simulink model "robotarm_A12"  (R2018b)
settings: Solver=FixedStepAuto  StartTime=0.0  StopTime=options.T_train  RelTol=1e-3  AbsTol=1e-6
undefined symbols (not defined in the file or in its folder): options
libraries: neural x132, simulink x2
(part 6 of 6)

== system robotarm_A12/NN_cex_1/Layer 3/Delays 1 ==
  "p{3}" : Inport  PortDimensions=30
      mask Display: e = 0.06;c1 = [120 230 180]/255;c2 = ([120 230 180]+0)/(256+128);c3 = ([120 230 180]+128)/(256+128);patch([0 1 1 0],[0 0 1 1],c1);patch([0 1 1 1-e 1-e 0+e],[0 0 1 1-e 0+e 0+e],c2);patch([0 0 1 1-e 0+e 0+e],[0 1 1 1-e 1-e 0+e],c3);plot([0 1 1 0 0],[0 0 1 1 0]);
  mux : Mux  Inputs=1
      mask Display: e = 0.06;c1 = [120 150 230]/255;c2 = ([120 150 230]+0)/383;c3 = ([120 150 230]+128)/383;patch([0 1 1 0],[0 0 1 1],c1);patch([0 1 1 1-e 1-e 0+e],[0 0 1 1-e 0+e 0+e],c2);patch([0 0 1 1-e 0+e 0+e],[0 1 1 1-e 1-e 0+e],c3);plot([0 1 1 0 0],[0 0 1 1 0]);disp('Mux')
  "pd{3,2}" : Outport
      mask Display: e = 0.06;c1 = [120 230 180]/255;c2 = ([120 230 180]+0)/(256+128);c3 = ([120 230 180]+128)/(256+128);patch([0 1 1 0],[0 0 1 1],c1);patch([0 1 1 1-e 1-e 0+e],[0 0 1 1-e 0+e 0+e],c2);patch([0 0 1 1-e 0+e 0+e],[0 1 1 1-e 1-e 0+e],c3);plot([0 1 1 0 0],[0 0 1 1 0]);
  wires:
  "p{3}"/1 -> mux/1
  mux/1 -> "pd{3,2}"/1

== system robotarm_A12/NN_cex_1/Layer 3/LW{3,2} ==
  "ad{3,2}" : Inport  PortDimensions=30
      mask Display: e = 0.06;c1 = [120 230 180]/255;c2 = ([120 230 180]+0)/(256+128);c3 = ([120 230 180]+128)/(256+128);patch([0 1 1 0],[0 0 1 1],c1);patch([0 1 1 1-e 1-e 0+e],[0 0 1 1-e 0+e 0+e],c2);patch([0 0 1 1-e 0+e 0+e],[0 1 1 1-e 1-e 0+e],c3);plot([0 1 1 0 0],[0 0 1 1 0]);
  "IW{3,2}(1,:)'" : Constant  Value=[0.73089943301855286872381611829041503369808197021484375;-0.53454468290774481697980036187800578773021697998046875;0.391308794320124331278520912746898829936981201171875;-0.035030971776598952838188694158816360868513584136962890625;-0.043214037250104538057104974768662941642105579376220703125;-0.217609448567078589409362621154286898672580718994140625;0.08874909364233929398579903136123903095722198486328125;0.414321294279813956418223597211181186139583587646484375;-0.006627272058408504619431145243879655026830732822418212890625;-0.2943870465255227220069400573265738785266876220703125;0.1833366258947856375360885294867330230772495269775390625;0.25722489727484276755831160699017345905303955078125;0.363800181621067364456934001282206736505031585693359375;0.499092008176059642732269594489480368793010711669921875;0.1578775111079609716480121051063179038465023040771484375;-0.75762710582779835277733582188375294208526611328125;0.218625137635059030305484384371084161102771759033203125;-0.0454027334397036630431188086731708608567714691162109375;-0.452458985302777116910277754868729971349239349365234375;-0.464402324168377622637393642435199581086635589599609375;-0.022425179128965112840266016291934647597372531890869140625;0.1678982785254042597866686037377803586423397064208984375;0.66287809285984466978192131136893294751644134521484375;0.266707022628045908874128144816495478153228759765625;-0.63508427839783931911910030976287089288234710693359375;0.363298042091588724300521562327048741281032562255859375;-0.07891971151895420255595325897957081906497478485107421875;0.256582107486141908214705154023249633610248565673828125;0.020925250491498674498824783540840144269168376922607421875;-0.423075256005668254299934005757677368819713592529296875]
      mask Display: e = 0.06;c1 = [120 150 230]/255;c2 = ([120 150 230]+0)/383;c3 = ([120 150 230]+128)/383;patch([0 1 1 0],[0 0 1 1],c1);patch([0 1 1 1-e 1-e 0+e],[0 0 1 1-e 0+e 0+e],c2);patch([0 0 1 1-e 0+e 0+e],[0 1 1 1-e 1-e 0+e],c3);plot([0 1 1 0 0],[0 0 1 1 0]);disp('weights');
  Mux : Mux  Inputs=1
      mask Display: e = 0.06;c1 = [120 150 230]/255;c2 = ([120 150 230]+0)/383;c3 = ([120 150 230]+128)/383;patch([0 1 1 0],[0 0 1 1],c1);patch([0 1 1 1-e 1-e 0+e],[0 0 1 1-e 0+e 0+e],c2);patch([0 0 1 1-e 0+e 0+e],[0 1 1 1-e 1-e 0+e],c3);plot([0 1 1 0 0],[0 0 1 1 0]);disp('Mux');
  dotprod1 : neural/Weight Functions/dotprod
  "lz{3,2}" : Outport
      mask Display: e = 0.06;c1 = [120 230 180]/255;c2 = ([120 230 180]+0)/(256+128);c3 = ([120 230 180]+128)/(256+128);patch([0 1 1 0],[0 0 1 1],c1);patch([0 1 1 1-e 1-e 0+e],[0 0 1 1-e 0+e 0+e],c2);patch([0 0 1 1-e 0+e 0+e],[0 1 1 1-e 1-e 0+e],c3);plot([0 1 1 0 0],[0 0 1 1 0]);
  wires:
  "IW{3,2}(1,:)'"/1 -> dotprod1/1
  "ad{3,2}"/1 -> dotprod1/2
  dotprod1/1 -> Mux/1
  Mux/1 -> "lz{3,2}"/1
